simulink library "INT_Tra_Add"  (R2016b)
settings: Solver=VariableStepAuto  StartTime=0.0  StopTime=10.0  RelTol=1e-3
settings Model: Creator=Administrator  LastModifiedBy=Administrator

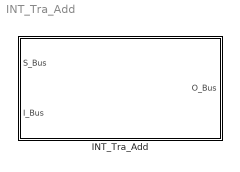
== system INT_Tra_Add ==
  INT_Tra_Add : Subsystem

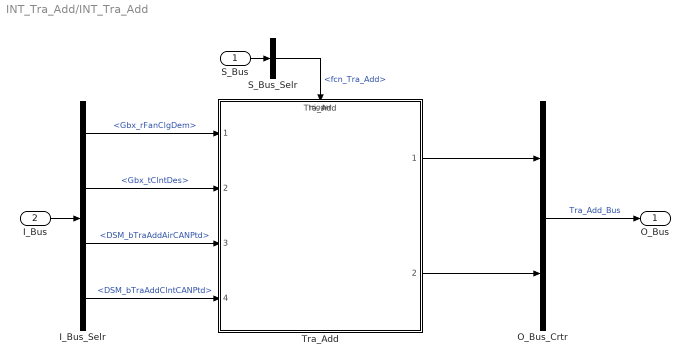
== system INT_Tra_Add/INT_Tra_Add ==
  S_Bus : Inport
  I_Bus : Inport  Port=2
  I_Bus_Selr : BusSelector  OutputSignals=Gbx_rFanClgDem,Gbx_tClntDes,DSM_bTraAddAirCANPtd,DSM_bTraAddClntCANPtd
  O_Bus_Crtr : BusCreator  Inputs=2
  S_Bus_Selr : BusSelector  OutputSignals=fcn_Tra_Add
  Tra_Add : ModelReference  ModelNameDialog=Tra_Add  SimulationMode=Normal  ModelReferenceVersion=1.13  TriggerPortName=function  TriggerPortTriggerType=function-call  TriggerPortStatesWhenEnabling=held
  O_Bus : Outport
  wires:
  S_Bus_Selr/1 -> Tra_Add/Trigger  "<fcn_Tra_Add>"
  S_Bus/1 -> S_Bus_Selr/1
  I_Bus/1 -> I_Bus_Selr/1
  I_Bus_Selr/1 -> Tra_Add/1  "<Gbx_rFanClgDem>"
  I_Bus_Selr/2 -> Tra_Add/2  "<Gbx_tClntDes>"
  I_Bus_Selr/3 -> Tra_Add/3  "<DSM_bTraAddAirCANPtd>"
  I_Bus_Selr/4 -> Tra_Add/4  "<DSM_bTraAddClntCANPtd>"
  O_Bus_Crtr/1 -> O_Bus/1  "Tra_Add_Bus"
  Tra_Add/1 -> O_Bus_Crtr/1
  Tra_Add/2 -> O_Bus_Crtr/2
